simulink model "flc"  (R2014a)
settings: Solver=ode45  StartTime=0.0  StopTime=10.0  RelTol=1e-3
undefined symbols (not defined in the file or in its folder): K
libraries: fuzblock x1
settings Model: Creator=krish  LastModifiedBy=KRISH

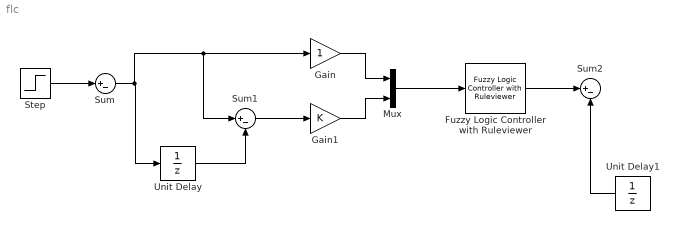
== system flc ==
  Fuzzy Logic Controller with Ruleviewer : fuzblock/Fuzzy Logic  Controller  with Ruleviewer  fismatrix=[]  Ts=2
  Gain : Gain
  Gain1 : Gain  Gain=K
  Mux : Mux  Inputs=2
  Step : Step  SampleTime=0
  Sum : Sum  Inputs=|+-
  Sum1 : Sum  Inputs=|+-
  Sum2 : Sum  Inputs=|+-
  Unit Delay : UnitDelay  SampleTime=-1
  Unit Delay1 : UnitDelay  SampleTime=-1
  wires:
  Mux/1 -> Fuzzy Logic Controller with Ruleviewer/1
  Sum/1 -> Sum1/1, Gain/1, Unit Delay/1
  Unit Delay/1 -> Sum1/2
  Sum1/1 -> Gain1/1
  Gain1/1 -> Mux/2
  Gain/1 -> Mux/1
  Step/1 -> Sum/1
  Fuzzy Logic Controller with Ruleviewer/1 -> Sum2/1
  Unit Delay1/1 -> Sum2/2
